simulink subsystem "Gsm_Subsystem"  (R2021b)
settings: Solver=VariableStepAuto  StartTime=0.0  StopTime=10.0  RelTol=1e-3
settings Model: Creator=levm1106  LastModifiedBy=sama1402

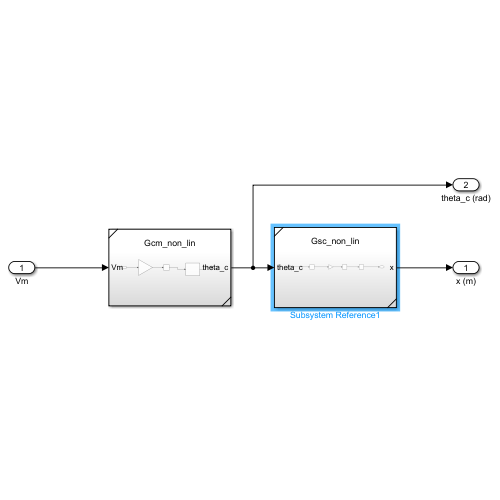
[thumbnail: Simulink's stored preview of the top-level diagram]
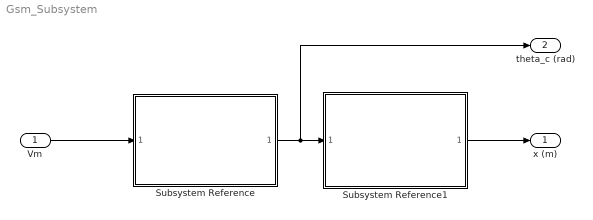
== system Gsm_Subsystem ==
  Vm : Inport
  Subsystem Reference : Subsystem  ReferencedSubsystem=Gcm_non_lin
  Subsystem Reference1 : Subsystem  ReferencedSubsystem=Gsc_non_lin
  x (m) : Outport
  theta_c (rad) : Outport  Port=2
  wires:
  Subsystem Reference1/1 -> x (m)/1
  Subsystem Reference/1 -> theta_c (rad)/1, Subsystem Reference1/1
  Vm/1 -> Subsystem Reference/1
